simulink model "smuling"  (R2018a)
settings: Solver=FixedStepDiscrete  StartTime=0.0  StopTime=100.0  FixedStep=10e-6  RelTol=1e-3
libraries: powerlib x2, re_lib x1
settings Model: Creator=IEK  LastModifiedBy=IEK

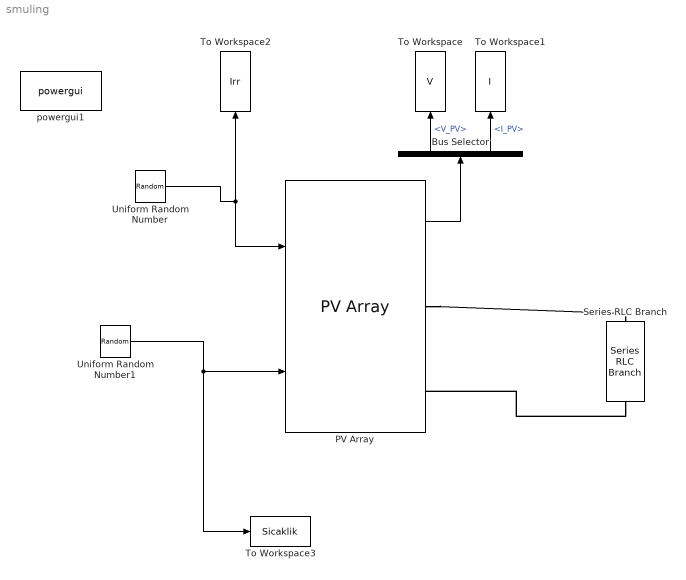
== system smuling ==
  Bus Selector : BusSelector  OutputSignals=V_PV,I_PV
  PV Array : re_lib/Solar/PV Array  Npar=3  Nser=8  PlotType=array @ 1000 W/m2 & specified temperatures  S_vec="[ 1000  500  100 ]"  Temp_C_vec="[ 45 25  ]"  ModuleName=1Soltech 1STH-215-P  PlotWhenSelected=off  Pm=213.15  Ncell=60  Voc=36.3  Isc=7.84  Vm=29  Im=7.35  beta_Voc_pc=-0.36099  alpha_Isc_pc=0.102  beta_Voc=-0.13104  alpha_Isc=0.007997  IL=7.8649  I0=2.9259e-10  nI=0.98117  Rsh=313.3991  Rs=0.39383  BAL=on  Tc=1e-6  Tfilter=5e-5
  Series RLC Branch : powerlib/Elements/Series RLC Branch  LConnTagsString=__new0  RConnTagsString=__new0  BranchType=R  Resistance=9.2  Inductance=1e-3  SetiL0=off  InitialCurrent=0  Capacitance=1e-6  Setx0=off  InitialVoltage=0  Measurements=None
  To Workspace : ToWorkspace  VariableName=V  SaveFormat=Timeseries  SampleTime=-1
  To Workspace1 : ToWorkspace  VariableName=I  SaveFormat=Timeseries  SampleTime=-1
  To Workspace2 : ToWorkspace  VariableName=Irr  SaveFormat=Timeseries  SampleTime=-1
  To Workspace3 : ToWorkspace  VariableName=Sicaklik  SaveFormat=Timeseries  SampleTime=-1
  Uniform Random Number : UniformRandomNumber  Minimum=750  Maximum=1000  SampleTime=0.1
  Uniform Random Number1 : UniformRandomNumber  Minimum=25  Maximum=45  SampleTime=0.1
  powergui1 : powerlib/powergui  Priority=1  SimulationMode=Discrete  SampleTime=0.1  frequency=60  Iterations=50  frequencyindice=0  Pbase=100e6  ErrMax=1e-4  UnitsV=kV  UnitsW=MW  buscounter=0  FunctionMessages=off  echomessages=off  EnableUseOfTLC=off  CurrentSourceSwitches=off  DisableSnubberDevices=off  DisableRonSwitches=off  DisableVfSwitches=off  DisplayEquations=off  SolverType=Tustin/Backward Euler (TBE)  Interpol=off  ExternalGateDelay=off  methode=off  Ts=100  x0status=blocks  SPID=on  SwTol=0  HookPort=off  RestoreLinks=warning  ResistiveCurrentMeasurement=off  Frange=[0:2:500]  Ylog=off  Xlog=on  ShowGrid=off  save=off  variable=ZData  structure=0  ZoomFFT=off  StartTime=0.0  cycles=1  DisplayStyle=1  fundamental=60  FreqAxis=off  MaxFrequency=1000  frequencyindicesteady=1  RmsSteady=1  display=off
  wires:
  Uniform Random Number1/1 -> To Workspace3/1, PV Array/2
  Uniform Random Number/1 -> To Workspace2/1, PV Array/1
  PV Array/1 -> Bus Selector/1
  Bus Selector/1 -> To Workspace/1  "<V_PV>"
  Bus Selector/2 -> To Workspace1/1  "<I_PV>"
  connections:
  PV Array/RConn1 -- Series RLC Branch/LConn1
  Series RLC Branch/RConn1 -- PV Array/RConn2
